simulink model "Earth"  (R2024b)
settings: Solver=VariableStepAuto  StartTime=0.0  StopTime=5e3  FixedStep=0.5  MaxStep=max_step_size  RelTol=1e-5
undefined symbols (not defined in the file): delta_t, Launch_site_vec, mu, omega, orbit_plane_normal, r_target, v_target
libraries: simulink_extras x1
settings Model: Creator=cpero  LastModifiedBy=cpero
settings SolverCC: MaxConsecutiveMinStep=1e6  EnableFixedStepZeroCrossing=on

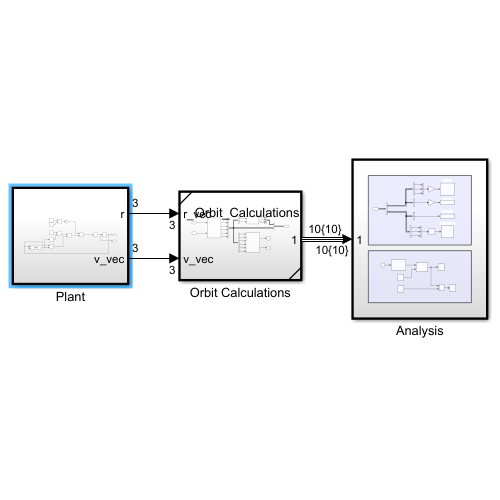
[thumbnail: Simulink's stored preview of the top-level diagram]
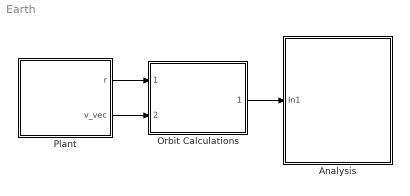
== system Earth ==
  Analysis : Subsystem
  Orbit Calculations : Subsystem  ReferencedSubsystem=Orbit_Calculations
  Plant : Subsystem
  wires:
  Orbit Calculations/1 -> Analysis/1(In1)
  Plant/1(r) -> Orbit Calculations/1
  Plant/2(v_vec) -> Orbit Calculations/2

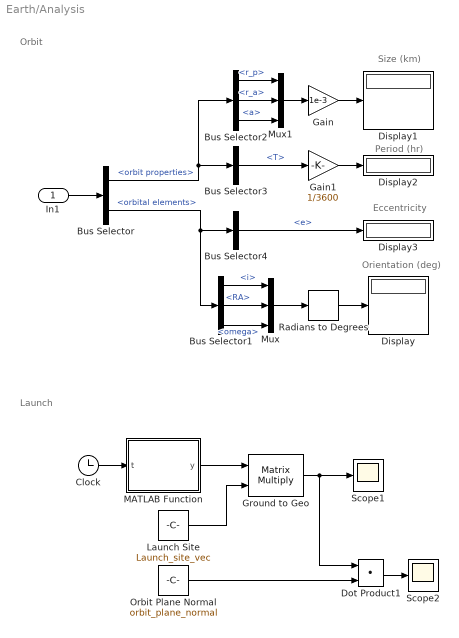
== system Earth/Analysis ==
  note: Launch
  note: Orbit
  note: Period (hr)
  note: Orientation (deg)
  note: Size (km)
  note: Eccentricity
  In1 : Inport
  Bus Selector : BusSelector  OutputSignals=orbit properties,orbital elements
  Bus Selector1 : BusSelector  OutputSignals=i,RA,omega
  Bus Selector2 : BusSelector  OutputSignals=r_p,r_a,a
  Bus Selector3 : BusSelector  OutputSignals=T
  Bus Selector4 : BusSelector  OutputSignals=e
  Clock : Clock
  Display{,1..3} (4 alike) : Display
  Dot Product1 : DotProduct  OutDataTypeStr=Inherit: Inherit via internal rule
  Gain : Gain  Gain=1e-3
  Gain1 : Gain  Gain=1/3600
  Ground to Geo : Product  Multiplication=Matrix(*)
  Launch Site : Constant  Value=Launch_site_vec
  MATLAB Function : MATLAB Function  TreatAsAtomicUnit=on
  Mux : Mux  Inputs=3
  Mux1 : Mux  Inputs=3
  Orbit Plane Normal : Constant  Value=orbit_plane_normal
  Radians to Degrees : simulink_extras/Transformations/Radians to Degrees
  Scope1 : Scope
  Scope2 : Scope
  wires:
  In1/1 -> Bus Selector/1
  Bus Selector/1 -> Bus Selector3/1, Bus Selector2/1  "<orbit properties>"
  Mux/1 -> Radians to Degrees/1
  Bus Selector/2 -> Bus Selector1/1, Bus Selector4/1  "<orbital elements>"
  Bus Selector1/1 -> Mux/1  "<i>"
  Bus Selector1/2 -> Mux/2  "<RA>"
  Radians to Degrees/1 -> Display/1
  Bus Selector1/3 -> Mux/3  "<omega>"
  Bus Selector2/1 -> Mux1/1  "<r_p>"
  Bus Selector2/2 -> Mux1/2  "<r_a>"
  Bus Selector2/3 -> Mux1/3  "<a>"
  Mux1/1 -> Gain/1
  Gain/1 -> Display1/1
  Bus Selector3/1 -> Gain1/1  "<T>"
  Gain1/1 -> Display2/1
  Bus Selector4/1 -> Display3/1  "<e>"
  Dot Product1/1 -> Scope2/1
  Orbit Plane Normal/1 -> Dot Product1/2
  Ground to Geo/1 -> Scope1/1, Dot Product1/1
  Clock/1 -> MATLAB Function/1(t)
  MATLAB Function/1(y) -> Ground to Geo/1
  Launch Site/1 -> Ground to Geo/2

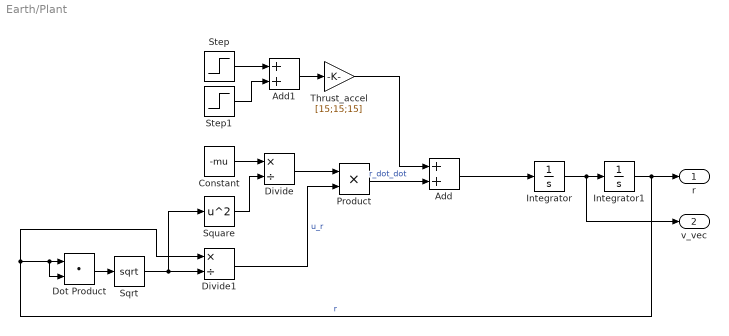
== system Earth/Plant ==
  Add : Sum
  Add1 : Sum
  Constant : Constant  Value=-mu
  Divide : Product  Inputs=*/
  Divide1 : Product  Inputs=*/
  Dot Product : DotProduct  OutDataTypeStr=Inherit: Inherit via internal rule
  Integrator : Integrator  InitialCondition=v_target
  Integrator1 : Integrator  InitialCondition=r_target
  Product : Product
  Sqrt : Sqrt
  Square : Math  Operator=square
  Step : Step  Time=1000  SampleTime=0
  Step1 : Step  Time=1001  After=-1  SampleTime=0
  Thrust_accel : Gain  Gain=[15;15;15]
  r : Outport
  v_vec : Outport  Port=2
  wires:
  Integrator1/1 -> Dot Product/2, Dot Product/1, Divide1/1, r/1  "r"
  Divide1/1 -> Product/2  "u_r"
  Sqrt/1 -> Square/1, Divide1/2
  Divide/1 -> Product/1
  Square/1 -> Divide/2
  Integrator/1 -> v_vec/1, Integrator1/1
  Dot Product/1 -> Sqrt/1
  Constant/1 -> Divide/1
  Add/1 -> Integrator/1
  Product/1 -> Add/2  "r_dot_dot"
  Step/1 -> Add1/1
  Step1/1 -> Add1/2
  Add1/1 -> Thrust_accel/1
  Thrust_accel/1 -> Add/1

== matlab function Earth/Analysis/MATLAB Function ==
  data: y output; t input; omega parameter; delta_t parameter
function y = fcn(t, omega, delta_t)
offset = delta_t;

y = [cos(omega*(t+offset)), -sin(omega*(t+offset)), 0;
     sin(omega*(t+offset)), cos(omega*(t+offset)), 0;
     0, 0, 1];
